simulink model "MPC_MG"  (R2020b)
settings: Solver=ode23tb  StartTime=0.0  StopTime=1  RelTol=1e-3
model workspace (MAT data in the model file):
  Ts = Simulink.Parameter
  Ts.Value = 5e-06
  Ts.DataType = 'auto'
  Ts.Dimensions = [1 1]
  secondary_on = Simulink.Parameter
  secondary_on.DataType = 'auto'
  secondary_on.Dimensions = [0 0]
values from neighbouring files (symbols this model uses):
  C_f = 50e-6    (= 5e-05)    [Four_DG_MG_PrimaryOnlyScript.m]    (also in MPC_MG_script.m; MPC_MG_script_raw_dmpc.m; MPC_MG_secondary_script.m; MPG_MG_July.m)
  f_c = 5000    [Four_DG_MG_PrimaryOnlyScript.m]    (also in MPC_MG_script.m = 40000; MPC_MG_script_raw_dmpc.m = 40000; MPC_MG_secondary_script.m = 40000; MPG_MG_July.m = 50000)
  kL = 1e-5    (= 1e-05)    [Four_DG_MG_PrimaryOnlyScript.m]    (also in MPC_MG_script.m = 1e-08; MPC_MG_script_raw_dmpc.m = 1e-08; MPC_MG_secondary_script.m = 1e-07; MPG_MG_July.m = 1e-07)
  L_f = 1.35e-3    (= 0.00135)    [Four_DG_MG_PrimaryOnlyScript.m]    (also in MPC_MG_script.m; MPC_MG_script_raw_dmpc.m; MPC_MG_secondary_script.m; MPG_MG_July.m)
  L_in1 = 0.35e-3    (= 0.00035)    [Four_DG_MG_PrimaryOnlyScript.m]    (also in MPC_MG_script.m; MPC_MG_script_raw_dmpc.m; MPC_MG_secondary_script.m; MPG_MG_July.m)
  L_in2 = 0.35e-3    (= 0.00035)    [Four_DG_MG_PrimaryOnlyScript.m]    (also in MPC_MG_script.m; MPC_MG_script_raw_dmpc.m; MPC_MG_secondary_script.m; MPG_MG_July.m)
  L_in3 = 0.35e-3    (= 0.00035)    [Four_DG_MG_PrimaryOnlyScript.m]    (also in MPC_MG_script.m; MPC_MG_script_raw_dmpc.m; MPC_MG_secondary_script.m; MPG_MG_July.m)
  L_in4 = 0.35e-3    (= 0.00035)    [Four_DG_MG_PrimaryOnlyScript.m]    (also in MPC_MG_script.m; MPC_MG_script_raw_dmpc.m; MPC_MG_secondary_script.m; MPG_MG_July.m)
  LD_ref1 = 800e-6    (= 0.0008)    [Four_DG_MG_PrimaryOnlyScript.m]    (also in MPC_MG_script.m = 0.0003; MPC_MG_script_raw_dmpc.m = 0.0003; MPC_MG_secondary_script.m = 0.0001; MPG_MG_July.m = 0.0004)
  lo_co = 0.2    [Four_DG_MG_PrimaryOnlyScript.m]    (also in MPC_MG_script.m = 0.05; MPC_MG_script_raw_dmpc.m; MPC_MG_secondary_script.m = 0.08; MPG_MG_July.m = 0.15)
  m_p1 = 9.4e-5/droopDivide    (= 9.4e-05)    [Four_DG_MG_PrimaryOnlyScript.m]    (also in MPC_MG_script.m; MPC_MG_script_raw_dmpc.m; MPC_MG_secondary_script.m; MPG_MG_July.m)
  m_p2 = 9.4e-5/droopDivide    (= 9.4e-05)    [Four_DG_MG_PrimaryOnlyScript.m]    (also in MPC_MG_script.m; MPC_MG_script_raw_dmpc.m; MPC_MG_secondary_script.m; MPG_MG_July.m)
  m_p3 = 12.5e-5/droopDivide    (= 0.000125)    [Four_DG_MG_PrimaryOnlyScript.m]    (also in MPC_MG_script.m; MPC_MG_script_raw_dmpc.m; MPC_MG_secondary_script.m; MPG_MG_July.m)
  m_p4 = 12.5e-5/droopDivide    (= 0.000125)    [Four_DG_MG_PrimaryOnlyScript.m]    (also in MPC_MG_script.m; MPC_MG_script_raw_dmpc.m; MPC_MG_secondary_script.m; MPG_MG_July.m)
  n_q1 = 1.3e-3/droopDivide2    (= 0.00013)    [Four_DG_MG_PrimaryOnlyScript.m]    (also in MPC_MG_script.m; MPC_MG_script_raw_dmpc.m; MPC_MG_secondary_script.m; MPG_MG_July.m)
  n_q2 = 1.3e-3/droopDivide2    (= 0.00013)    [Four_DG_MG_PrimaryOnlyScript.m]    (also in MPC_MG_script.m; MPC_MG_script_raw_dmpc.m; MPC_MG_secondary_script.m; MPG_MG_July.m)
  n_q3 = 1.5e-3/droopDivide2    (= 0.00015)    [Four_DG_MG_PrimaryOnlyScript.m]    (also in MPC_MG_script.m; MPC_MG_script_raw_dmpc.m; MPC_MG_secondary_script.m; MPG_MG_July.m)
  n_q4 = 1.5e-3/droopDivide2    (= 0.00015)    [Four_DG_MG_PrimaryOnlyScript.m]    (also in MPC_MG_script.m; MPC_MG_script_raw_dmpc.m; MPC_MG_secondary_script.m; MPG_MG_July.m)
  R_f = 0.1    [Four_DG_MG_PrimaryOnlyScript.m]    (also in MPC_MG_script.m; MPC_MG_script_raw_dmpc.m; MPC_MG_secondary_script.m; MPG_MG_July.m)
  R_in1 = 0.03    [Four_DG_MG_PrimaryOnlyScript.m]    (also in MPC_MG_script.m; MPC_MG_script_raw_dmpc.m; MPC_MG_secondary_script.m; MPG_MG_July.m)
  R_in2 = 0.03    [Four_DG_MG_PrimaryOnlyScript.m]    (also in MPC_MG_script.m; MPC_MG_script_raw_dmpc.m; MPC_MG_secondary_script.m; MPG_MG_July.m)
  R_in3 = 0.03    [Four_DG_MG_PrimaryOnlyScript.m]    (also in MPC_MG_script.m; MPC_MG_script_raw_dmpc.m; MPC_MG_secondary_script.m; MPG_MG_July.m)
  R_in4 = 0.03    [Four_DG_MG_PrimaryOnlyScript.m]    (also in MPC_MG_script.m; MPC_MG_script_raw_dmpc.m; MPC_MG_secondary_script.m; MPG_MG_July.m)
  Ts = 10e-6    (= 1e-05)    [Four_DG_MG_PrimaryOnlyScript.m]    (also in MPC_MG_script.m; MPC_MG_script_raw_dmpc.m; MPC_MG_secondary_script.m; MPG_MG_July.m)
  V_nom = 220*sqrt(2)    [Four_DG_MG_PrimaryOnlyScript.m]    (also in MPC_MG_script.m; MPC_MG_script_raw_dmpc.m; MPC_MG_secondary_script.m; MPG_MG_July.m)
  Vdc = 600    [Four_DG_MG_PrimaryOnlyScript.m]    (also in MPC_MG_script.m; MPC_MG_script_raw_dmpc.m; MPC_MG_secondary_script.m; MPG_MG_July.m)
  w_c_high = 2*pi*50    (= 314.159265359)    [Four_DG_MG_PrimaryOnlyScript.m]    (also in MPC_MG_script.m; MPC_MG_script_raw_dmpc.m; MPC_MG_secondary_script.m; MPG_MG_July.m)
  w_nom = 2*pi*50    (= 314.159265359)    [Four_DG_MG_PrimaryOnlyScript.m]    (also in MPC_MG_script.m; MPC_MG_script_raw_dmpc.m; MPC_MG_secondary_script.m; MPG_MG_July.m)
undefined symbols (not defined in the file or in its folder): i
libraries: powerlib x53, powerlib_meascontrol x19, eeGeneralControl x10, dspswit3 x5
(part 1 of 3)
settings Model: SimulationMode=accelerator  Creator=Linh  LastModifiedBy=Linh
settings DataIOCC: ReturnWorkspaceOutputs=off

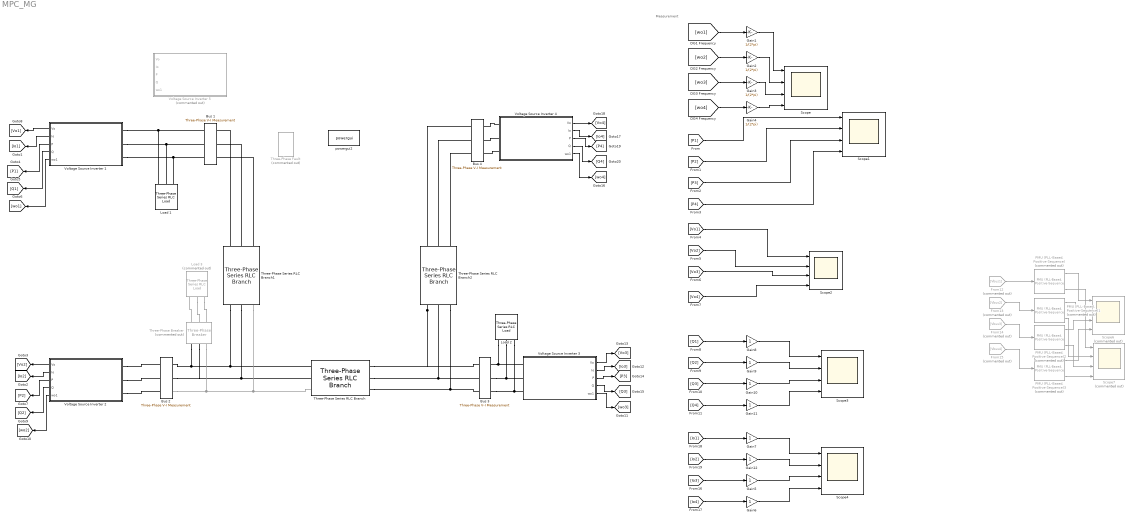
== system MPC_MG ==
  note: Measurement
  Bus 1 : powerlib/Measurements/Three-Phase V-I Measurement  VoltageMeasurement=phase-to-ground  SetLabelV=on  LabelV=Vbus1  Vpu=on  VpuLL=off  CurrentMeasurement=yes  SetLabelI=on  LabelI=Ibus1  Ipu=off  Pbase=100e6  Vbase=380  OutputType=Complex  PhasorSimulation=off  PSBequivalent=0
  Bus 2 : powerlib/Measurements/Three-Phase V-I Measurement  VoltageMeasurement=phase-to-ground  SetLabelV=on  LabelV=Vbus2  Vpu=on  VpuLL=off  CurrentMeasurement=yes  SetLabelI=on  LabelI=Ibus2  Ipu=off  Pbase=100e6  Vbase=380  OutputType=Complex  PhasorSimulation=off  PSBequivalent=0
  Bus 3 : powerlib/Measurements/Three-Phase V-I Measurement  VoltageMeasurement=phase-to-ground  SetLabelV=on  LabelV=Vbus3  Vpu=on  VpuLL=off  CurrentMeasurement=yes  SetLabelI=on  LabelI=Ibus3  Ipu=off  Pbase=100e6  Vbase=380  OutputType=Complex  PhasorSimulation=off  PSBequivalent=0
  Bus 4 : powerlib/Measurements/Three-Phase V-I Measurement  VoltageMeasurement=phase-to-phase  SetLabelV=on  LabelV=Vbus4  Vpu=off  VpuLL=on  CurrentMeasurement=no  SetLabelI=off  LabelI=Ibus4  Ipu=off  Pbase=100e6  Vbase=380  OutputType=Complex  PhasorSimulation=off  PSBequivalent=0
  From12 : From  Commented=on  GotoTag=Vbus1  TagVisibility=global
  From13 : From  Commented=on  GotoTag=Vbus2  TagVisibility=global
  From14 : From  Commented=on  GotoTag=Vbus3  TagVisibility=global
  From15 : From  Commented=on  GotoTag=Vbus4  TagVisibility=global
  Gain{1..4} (4 alike) : Gain  Gain=1/(2*pi)
  Gain{5..12} (8 alike) : Gain
  Load 1 : powerlib/Elements/Three-Phase Series RLC Load  LConnTagsString=A|B|C  Configuration=Y (grounded)  NominalVoltage=220*sqrt(3)  Vabc=[1e3 1e3 1e3]  Vabcp=[1e3 1e3 1e3]  NominalFrequency=50  UnbalancedPower=off  ActivePower=12000*3  InductivePower=12000*3  CapacitivePower=0  Pabc=[10e3 9e3 11e3]  QLabc=[100 90 110]  QCabc=[100 90 110]  Pabcp=[10e3 9e3 11e3]  QLabcp=[100 90 110]  QCabcp=[100 90 110]  Measurements=Branch voltages and currents  LoadType=constant Z
  Load 2 : powerlib/Elements/Three-Phase Series RLC Load  LConnTagsString=A|B|C  Configuration=Y (grounded)  NominalVoltage=220*sqrt(3)  Vabc=[1e3 1e3 1e3]  Vabcp=[1e3 1e3 1e3]  NominalFrequency=50  UnbalancedPower=off  ActivePower=15300*3  InductivePower=7600*3  CapacitivePower=0  Pabc=[10e3 9e3 11e3]  QLabc=[100 90 110]  QCabc=[100 90 110]  Pabcp=[10e3 9e3 11e3]  QLabcp=[100 90 110]  QCabcp=[100 90 110]  Measurements=Branch voltages and currents  LoadType=constant Z
  Load 3 : powerlib/Elements/Three-Phase Series RLC Load  Commented=on  LConnTagsString=A|B|C  Configuration=Y (grounded)  NominalVoltage=220*sqrt(3)  Vabc=[1e3 1e3 1e3]  Vabcp=[1e3 1e3 1e3]  NominalFrequency=50  UnbalancedPower=off  ActivePower=20000*3  InductivePower=12000*3  CapacitivePower=0  Pabc=[10e3 9e3 11e3]  QLabc=[100 90 110]  QCabc=[100 90 110]  Pabcp=[10e3 9e3 11e3]  QLabcp=[100 90 110]  QCabcp=[100 90 110]  Measurements=Branch voltages and currents  LoadType=constant Z
  PMU (PLL-Based, Positive-Sequence){,1..3} (4 alike) : powerlib_meascontrol/Measurements/PMU (PLL-Based, Positive-Sequence)  Commented=on  nominalFrequency=50  samplingRate=64  reportingFactor=5
      settings: SourceProductBaseCode=PS
  Scope{,1..4} (5 alike) : Scope  NumInputPorts=4
  Scope6 : Scope  Commented=on  NumInputPorts=4
  Scope7 : Scope  Commented=on  NumInputPorts=4
  Three-Phase Series RLC Branch : powerlib/Elements/Three-Phase Series RLC Branch  LConnTagsString=A|B|C  RConnTagsString=A|B|C  BranchType=RL  Resistance=0.35  Inductance=1847e-6  Capacitance=1e-6  Measurements=Branch voltages and currents
  Three-Phase Series RLC Branch1 : powerlib/Elements/Three-Phase Series RLC Branch  LConnTagsString=A|B|C  RConnTagsString=A|B|C  BranchType=RL  Resistance=0.23  Inductance=318e-6  Capacitance=1e-6  Measurements=Branch voltages and currents
  Three-Phase Series RLC Branch2 : powerlib/Elements/Three-Phase Series RLC Branch  LConnTagsString=A|B|C  RConnTagsString=A|B|C  BranchType=RL  Resistance=0.23  Inductance=318e-6  Capacitance=1e-6  Measurements=Branch voltages and currents
  Three-Phase Breaker : powerlib/Elements/Three-Phase Breaker  Commented=on  InitialState=open  SwitchA=on  SwitchB=on  SwitchC=on  SwitchTimes="[0.5  2]"  External=off  BreakerResistance=0.01  SnubberResistance=1e6  SnubberCapacitance=inf  Measurements=None
  Three-Phase Fault : powerlib/Elements/Three-Phase Fault  Commented=on  InitialStates=0  FaultA=on  FaultB=on  FaultC=off  GroundFault=off  SwitchTimes="[0.2  0.24]"  External=off  SwitchStatus=NaN  FaultResistance=0.001  GroundResistance=0.01  SnubberResistance=1e6  SnubberCapacitance=inf  Measurements=None
  Voltage Source Inverter 1 : Subsystem  mask{w_nom=w_nom, V_nom=V_nom, modT=1/f_c, m_p=m_p1, n_q=n_q1, LD_ref=LD_ref1, k_LD=kL, w_c_high=[1 w_c_high], R_f=R_f, L_f=L_f, C_f=C_f, R_in=R_in1, L_in=L_in1}
      mask prompts: w_nom "Nominal frequency (radian)"; V_nom "Nominal voltage"; modT "Sampling Time"; m_p "P-w gain"; n_q "Q-V gain"; LD_ref "Reference virtual impedance (H)"; k_LD "Virtual impedance Q gain"; w_c_high "High-pass filter denominator:"; R_f "Inductor resistance:"; L_f "Filter inductance"; C_f "Filter capacitance"; R_in "Resistance coupling"; L_in "Inductance coupling"
      mask TypeOptions w_nom: w_nom/Value
      mask TypeOptions V_nom: V_nom/Value
      mask TypeOptions modT:
      | Model Predictive Control
      | /Ts
      mask TypeOptions m_p: Droop for secondary control2/Gain5/Gain
      mask TypeOptions n_q: Droop for secondary control2/Gain4/Gain
      mask TypeOptions LD_ref: LD_ref/Value
      mask TypeOptions k_LD: k_LD/Gain
      mask TypeOptions w_c_high: High-Pass Filter/Denominator
      mask TypeOptions R_f:
      | Three-Phase
      | Series RLC Branch/Resistance
      mask TypeOptions L_f:
      | Three-Phase
      | Series RLC Branch/Inductance
      mask TypeOptions C_f:
      | Three-Phase
      | Series RLC Branch2/Capacitance
      mask TypeOptions R_in:
      | Three-Phase
      | Series RLC Branch1/Resistance
      mask TypeOptions L_in:
      | Three-Phase
      | Series RLC Branch1/Inductance
      mask DialogControl ParameterGroupVar Prompt: Microgrid-wide values
      mask DialogControl Container5 Prompt: Droop value
      mask DialogControl Container8 Prompt: Filter
  Voltage Source Inverter 2 : Subsystem  mask{w_nom=w_nom, V_nom=V_nom, modT=1/f_c, m_p=m_p2, n_q=n_q2, LD_ref=LD_ref1, k_LD=kL, w_c_high=[1 w_c_high], R_f=R_f, L_f=L_f, C_f=C_f, R_in=R_in2, L_in=L_in2}
      mask prompts: w_nom "Nominal frequency (radian)"; V_nom "Nominal voltage"; modT "Sampling Time"; m_p "P-w gain"; n_q "Q-V gain"; LD_ref "Reference virtual impedance (H)"; k_LD "Virtual impedance Q gain"; w_c_high "High-pass filter denominator:"; R_f "Inductor resistance:"; L_f "Filter inductance"; C_f "Filter capacitance"; R_in "Resistance coupling"; L_in "Inductance coupling"
      mask TypeOptions w_nom: w_nom/Value
      mask TypeOptions V_nom: V_nom/Value
      mask TypeOptions modT:
      | Model Predictive Control
      | /Ts
      mask TypeOptions m_p: Droop for secondary control2/Gain5/Gain
      mask TypeOptions n_q: Droop for secondary control2/Gain4/Gain
      mask TypeOptions LD_ref: LD_ref/Value
      mask TypeOptions k_LD: k_LD/Gain
      mask TypeOptions w_c_high: High-Pass Filter/Denominator
      mask TypeOptions R_f:
      | Three-Phase
      | Series RLC Branch/Resistance
      mask TypeOptions L_f:
      | Three-Phase
      | Series RLC Branch/Inductance
      mask TypeOptions C_f:
      | Three-Phase
      | Series RLC Branch2/Capacitance
      mask TypeOptions R_in:
      | Three-Phase
      | Series RLC Branch1/Resistance
      mask TypeOptions L_in:
      | Three-Phase
      | Series RLC Branch1/Inductance
      mask DialogControl ParameterGroupVar Prompt: Microgrid-wide values
      mask DialogControl Container5 Prompt: Droop value
      mask DialogControl Container8 Prompt: Filter
  Voltage Source Inverter 3 : Subsystem  mask{w_nom=w_nom, V_nom=V_nom, modT=1/f_c, m_p=m_p3, n_q=n_q3, LD_ref=LD_ref1, k_LD=kL, w_c_high=[1 w_c_high], R_f=R_f, L_f=L_f, C_f=C_f, R_in=R_in3, L_in=L_in3}
      mask prompts: w_nom "Nominal frequency (radian)"; V_nom "Nominal voltage"; modT "Sampling Time"; m_p "P-w gain"; n_q "Q-V gain"; LD_ref "Reference virtual impedance (H)"; k_LD "Virtual impedance Q gain"; w_c_high "High-pass filter denominator:"; R_f "Inductor resistance:"; L_f "Filter inductance"; C_f "Filter capacitance"; R_in "Resistance coupling"; L_in "Inductance coupling"
      mask TypeOptions w_nom: w_nom/Value
      mask TypeOptions V_nom: V_nom/Value
      mask TypeOptions modT:
      | Model Predictive Control
      | /Ts
      mask TypeOptions m_p: Droop for secondary control2/Gain5/Gain
      mask TypeOptions n_q: Droop for secondary control2/Gain4/Gain
      mask TypeOptions LD_ref: LD_ref/Value
      mask TypeOptions k_LD: k_LD/Gain
      mask TypeOptions w_c_high: High-Pass Filter/Denominator
      mask TypeOptions R_f:
      | Three-Phase
      | Series RLC Branch/Resistance
      mask TypeOptions L_f:
      | Three-Phase
      | Series RLC Branch/Inductance
      mask TypeOptions C_f:
      | Three-Phase
      | Series RLC Branch2/Capacitance
      mask TypeOptions R_in:
      | Three-Phase
      | Series RLC Branch1/Resistance
      mask TypeOptions L_in:
      | Three-Phase
      | Series RLC Branch1/Inductance
      mask DialogControl ParameterGroupVar Prompt: Microgrid-wide values
      mask DialogControl Container5 Prompt: Droop value
      mask DialogControl Container8 Prompt: Filter
  Voltage Source Inverter 4 : Subsystem  mask{w_nom=w_nom, V_nom=V_nom, modT=1/f_c, m_p=m_p4, n_q=n_q4, LD_ref=LD_ref1, k_LD=kL, w_c_high=[1 w_c_high], R_f=R_f, L_f=L_f, C_f=C_f, R_in=R_in4, L_in=L_in4}
      mask prompts: w_nom "Nominal frequency (radian)"; V_nom "Nominal voltage"; modT "Sampling Time"; m_p "P-w gain"; n_q "Q-V gain"; LD_ref "Reference virtual impedance (H)"; k_LD "Virtual impedance Q gain"; w_c_high "High-pass filter denominator:"; R_f "Inductor resistance:"; L_f "Filter inductance"; C_f "Filter capacitance"; R_in "Resistance coupling"; L_in "Inductance coupling"
      mask TypeOptions w_nom: w_nom/Value
      mask TypeOptions V_nom: V_nom/Value
      mask TypeOptions modT:
      | Model Predictive Control
      | /Ts
      mask TypeOptions m_p: Droop for secondary control2/Gain5/Gain
      mask TypeOptions n_q: Droop for secondary control2/Gain4/Gain
      mask TypeOptions LD_ref: LD_ref/Value
      mask TypeOptions k_LD: k_LD/Gain
      mask TypeOptions w_c_high: High-Pass Filter/Denominator
      mask TypeOptions R_f:
      | Three-Phase
      | Series RLC Branch/Resistance
      mask TypeOptions L_f:
      | Three-Phase
      | Series RLC Branch/Inductance
      mask TypeOptions C_f:
      | Three-Phase
      | Series RLC Branch2/Capacitance
      mask TypeOptions R_in:
      | Three-Phase
      | Series RLC Branch1/Resistance
      mask TypeOptions L_in:
      | Three-Phase
      | Series RLC Branch1/Inductance
      mask DialogControl ParameterGroupVar Prompt: Microgrid-wide values
      mask DialogControl Container5 Prompt: Droop value
      mask DialogControl Container8 Prompt: Filter
  Voltage Source Inverter 5 : Subsystem  Commented=on  mask{w_nom=w_nom, V_nom=V_nom, modT=1/f_c, m_p=m_p1, n_q=n_q1, LD_ref=LD_ref1, k_LD=kL, w_c_high=[1 w_c_high], R_f=R_f, L_f=L_f, C_f=C_f, R_in=R_in1, L_in=L_in1}
      mask prompts: w_nom "Nominal frequency (radian)"; V_nom "Nominal voltage"; modT "Sampling Time"; m_p "P-w gain"; n_q "Q-V gain"; LD_ref "Reference virtual impedance (H)"; k_LD "Virtual impedance Q gain"; w_c_high "High-pass filter denominator:"; R_f "Inductor resistance:"; L_f "Filter inductance"; C_f "Filter capacitance"; R_in "Resistance coupling"; L_in "Inductance coupling"
      mask TypeOptions w_nom: w_nom/Value
      mask TypeOptions V_nom: V_nom/Value
      mask TypeOptions modT:
      | Model Predictive Control
      | /Ts
      mask TypeOptions m_p: Droop for secondary control2/Gain5/Gain
      mask TypeOptions n_q: Droop for secondary control2/Gain4/Gain
      mask TypeOptions LD_ref: LD_ref/Value
      mask TypeOptions k_LD: k_LD/Gain
      mask TypeOptions w_c_high: High-Pass Filter/Denominator
      mask TypeOptions R_f:
      | Three-Phase
      | Series RLC Branch/Resistance
      mask TypeOptions L_f:
      | Three-Phase
      | Series RLC Branch/Inductance
      mask TypeOptions C_f:
      | Three-Phase
      | Series RLC Branch2/Capacitance
      mask TypeOptions R_in:
      | Three-Phase
      | Series RLC Branch1/Resistance
      mask TypeOptions L_in:
      | Three-Phase
      | Series RLC Branch1/Inductance
      mask DialogControl ParameterGroupVar Prompt: Microgrid-wide values
      mask DialogControl Container5 Prompt: Droop value
      mask DialogControl Container8 Prompt: Filter
  powergui2 : powerlib/powergui  Priority=1  SimulationMode=Discrete  SampleTime=Ts  frequency=60  Iterations=50  frequencyindice=0  Pbase=100e6  ErrMax=1e-4  UnitsV=kV  UnitsW=MW  buscounter=0  FunctionMessages=off  echomessages=off  EnableUseOfTLC=off  CurrentSourceSwitches=off  DisableSnubberDevices=off  DisableRonSwitches=off  DisableVfSwitches=off  DisplayEquations=off  AutomaticDiscreteSolvers=off  SolverType=Tustin/Backward Euler (TBE)  Interpol=off  ExternalGateDelay=off  methode=off  Ts=100  x0status=blocks  SPID=on  SwTol=0  HookPort=off  NonlinearTolerance=1e-4  nMaxIteration=100  ContinueOnMaxIteration=off  RestoreLinks=warning  ResistiveCurrentMeasurement=off  Frange=[0:2:500]  Ylog=off  Xlog=on  ShowGrid=off  save=off  variable=ZData  structure=ScopeData3  ZoomFFT=off  StartTime=0.5  cycles=1  DisplayStyle=1  fundamental=50  FreqAxis=off  MaxFrequency=1000  frequencyindicesteady=1  RmsSteady=1  display=off
  wires:
  Voltage Source Inverter 1/1(Vo) -> [Vo1]
  Voltage Source Inverter 1/2(Io) -> [Io1]
  Voltage Source Inverter 2/1(Vo) -> [Vo2]
  Voltage Source Inverter 2/2(Io) -> [Io2]
  Voltage Source Inverter 1/3(P) -> [P1]
  Voltage Source Inverter 1/4(Q) -> [Q1]
  Voltage Source Inverter 1/5(wo1) -> [wo1]
  Voltage Source Inverter 2/3(P) -> [P2]
  Voltage Source Inverter 2/4(Q) -> [Q2]
  Voltage Source Inverter 2/5(wo1) -> [wo2]
  Voltage Source Inverter 3/5(wo1) -> [wo3]
  Voltage Source Inverter 3/3(P) -> [P3]
  Voltage Source Inverter 3/1(Vo) -> [Vo3]
  Voltage Source Inverter 3/4(Q) -> [Q3]
  Voltage Source Inverter 3/2(Io) -> [Io3]
  Voltage Source Inverter 4/2(Io) -> [Io4]
  Voltage Source Inverter 4/5(wo1) -> [wo4]
  Voltage Source Inverter 4/1(Vo) -> [Vo4]
  Voltage Source Inverter 4/4(Q) -> [Q4]
  Voltage Source Inverter 4/3(P) -> [P4]
  "PMU (PLL-Based, Positive-Sequence)1"/3 -> Scope7/2
  From12/1 -> "PMU (PLL-Based, Positive-Sequence)"/1
  Gain8/1 -> Scope3/1
  Gain11/1 -> Scope3/4
  [Q4] -> Gain11/1
  [Q1] -> Gain8/1
  [wo3] -> Gain3/1
  "PMU (PLL-Based, Positive-Sequence)3"/1 -> Scope6/4
  Gain2/1 -> Scope/2
  Gain4/1 -> Scope/4
  "PMU (PLL-Based, Positive-Sequence)2"/3 -> Scope7/3
  [wo1] -> Gain1/1
  "PMU (PLL-Based, Positive-Sequence)2"/1 -> Scope6/3
  From14/1 -> "PMU (PLL-Based, Positive-Sequence)2"/1
  [P1] -> Scope1/1
  "PMU (PLL-Based, Positive-Sequence)3"/3 -> Scope7/4
  "PMU (PLL-Based, Positive-Sequence)"/1 -> Scope6/1
  "PMU (PLL-Based, Positive-Sequence)"/3 -> Scope7/1
  "PMU (PLL-Based, Positive-Sequence)1"/1 -> Scope6/2
  From13/1 -> "PMU (PLL-Based, Positive-Sequence)1"/1
  [Vo4] -> Scope2/4
  [P3] -> Scope1/3
  [Q2] -> Gain9/1
  Gain9/1 -> Scope3/2
  [P2] -> Scope1/2
  Gain3/1 -> Scope/3
  [Vo2] -> Scope2/2
  [Vo3] -> Scope2/3
  [Vo1] -> Scope2/1
  [wo2] -> Gain2/1
  [Q3] -> Gain10/1
  Gain1/1 -> Scope/1
  [P4] -> Scope1/4
  Gain10/1 -> Scope3/3
  From15/1 -> "PMU (PLL-Based, Positive-Sequence)3"/1
  [wo4] -> Gain4/1
  [Io3] -> Gain5/1
  [Io1] -> Gain7/1
  [Io2] -> Gain12/1
  Gain6/1 -> Scope4/4
  [Io4] -> Gain6/1
  Gain5/1 -> Scope4/3
  Gain7/1 -> Scope4/1
  Gain12/1 -> Scope4/2
  connections:
  Voltage Source Inverter 2/LConn1 -- Bus 2/LConn1
  Voltage Source Inverter 2/LConn2 -- Bus 2/LConn2
  Voltage Source Inverter 2/LConn3 -- Bus 2/LConn3
  Three-Phase Series RLC Branch1/RConn2 -- Three-Phase Series RLC Branch/LConn2 -- Three-Phase Breaker/LConn2 -- Bus 2/RConn2
  Bus 3/LConn2 -- Three-Phase Series RLC Branch/RConn2 -- Three-Phase Series RLC Branch2/RConn2
  Load 1/LConn3 -- Voltage Source Inverter 1/LConn3 -- Bus 1/LConn3
  Bus 2/RConn1 -- Three-Phase Series RLC Branch/LConn1 -- Three-Phase Series RLC Branch1/RConn1 -- Three-Phase Breaker/LConn1
  Three-Phase Breaker/LConn3 -- Three-Phase Series RLC Branch/LConn3 -- Three-Phase Series RLC Branch1/RConn3 -- Bus 2/RConn3
  Load 2/LConn2 -- Voltage Source Inverter 3/LConn2 -- Bus 3/RConn2
  Bus 3/LConn3 -- Three-Phase Series RLC Branch/RConn3 -- Three-Phase Series RLC Branch2/RConn3
  Load 2/LConn1 -- Voltage Source Inverter 3/LConn1 -- Bus 3/RConn1
  Load 1/LConn2 -- Voltage Source Inverter 1/LConn2 -- Bus 1/LConn2
  Three-Phase Series RLC Branch2/RConn1 -- Three-Phase Series RLC Branch/RConn1 -- Bus 3/LConn1
  Load 2/LConn3 -- Voltage Source Inverter 3/LConn3 -- Bus 3/RConn3
  Load 1/LConn1 -- Voltage Source Inverter 1/LConn1 -- Bus 1/LConn1
  Three-Phase Series RLC Branch1/LConn2 -- Bus 1/RConn2
  Load 3/LConn3 -- Three-Phase Breaker/RConn3
  Three-Phase Series RLC Branch2/LConn1 -- Bus 4/LConn1
  Three-Phase Breaker/RConn1 -- Load 3/LConn1
  Three-Phase Series RLC Branch1/LConn1 -- Bus 1/RConn1
  Three-Phase Series RLC Branch2/LConn3 -- Bus 4/LConn3
  Three-Phase Series RLC Branch2/LConn2 -- Bus 4/LConn2
  Three-Phase Series RLC Branch1/LConn3 -- Bus 1/RConn3
  Load 3/LConn2 -- Three-Phase Breaker/RConn2
  Voltage Source Inverter 4/LConn1 -- Bus 4/RConn1
  Voltage Source Inverter 4/LConn2 -- Bus 4/RConn2
  Voltage Source Inverter 4/LConn3 -- Bus 4/RConn3

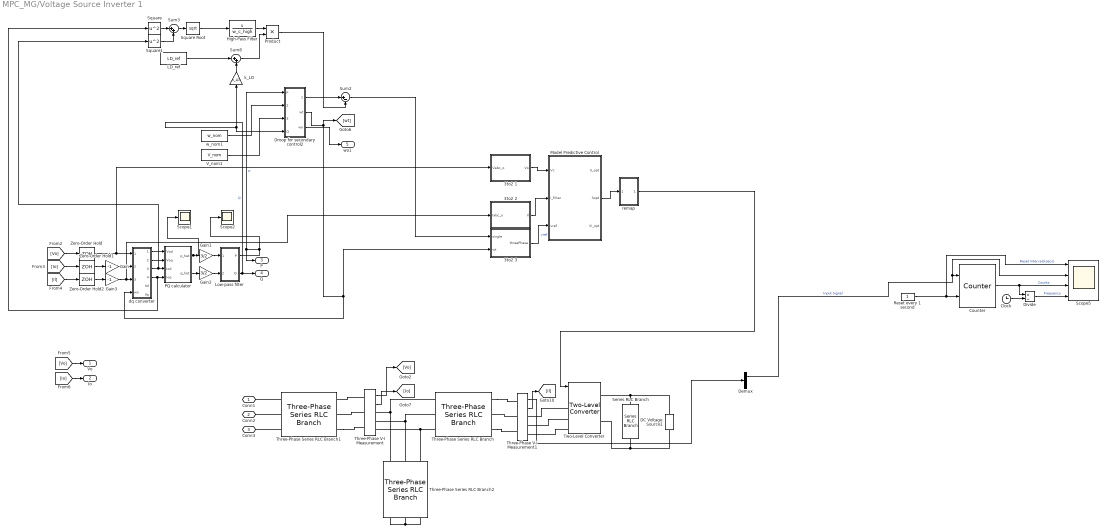
== system MPC_MG/Voltage Source Inverter 1 ==
  3to2 1 : Subsystem
  3to2 2 : Subsystem
  3to2 3 : Subsystem
  Clock : Clock
  Counter : dspswit3/Counter  Direction=Up  CountEvent=Rising edge  CounterSize=User defined  MaxCount=5e5  InitialCount=0  Output=Count  HitValue=1  ResetInput=on  SamplesPerFrame=1  Ts=1  CntDtype=double  HitDtype=Logical
  DC Voltage Source1 : powerlib/Electrical Sources/DC Voltage Source  Amplitude=Vdc  Measurements=None
  Demux : Demux  Outputs=3
  Divide : Product  Inputs=*/
  Droop for secondary control2 : Subsystem
  Gain : Gain  Gain=-1
  Gain1 : Gain  Gain=3/2
  Gain2 : Gain  Gain=3/2
  Gain3 : Gain  Gain=-1
  High-Pass Filter : TransferFcn  Numerator=[1 0]  Denominator=w_c_high
  LD_ref : Constant  Value=LD_ref
  Low-pass filter : Subsystem
  "Model Predictive Control " : MATLAB Function  TreatAsAtomicUnit=on  mask{Ts=modT, Cfilter=C_f, Lfilter=L_f, Vdc=Vdc}
      mask prompts: Ts "Sampling Time"; Cfilter "Filter Capacitor"; Lfilter "Filter Inductance"; Vdc "Input DC Voltage"
  PQ calculator : Subsystem
  Product : Product
  Reset every 1 second : Constant
  Scope1 : Scope
  Scope2 : Scope
  Scope5 : Scope  NumInputPorts=4
  Series RLC Branch : powerlib/Elements/Series RLC Branch  LConnTagsString=__new0  RConnTagsString=__new0  BranchType=RC  Resistance=30  Inductance=1e-3  SetiL0=off  InitialCurrent=0  Capacitance=80e-6  Setx0=off  InitialVoltage=0  Measurements=None
  Square : Math  Operator=square  SaturateOnIntegerOverflow=on
  Square Root : Sqrt  SaturateOnIntegerOverflow=on
  Square1 : Math  Operator=square  SaturateOnIntegerOverflow=on
  Sum2 : Sum  Inputs=|+-
  Sum3 : Sum  Inputs=|++
  Sum8 : Sum  Inputs=|++
  Three-Phase Series RLC Branch : powerlib/Elements/Three-Phase Series RLC Branch  LConnTagsString=A|B|C  RConnTagsString=A|B|C  BranchType=RL  Resistance=R_f  Inductance=L_f  Capacitance=1e-6  Measurements=None
  Three-Phase Series RLC Branch1 : powerlib/Elements/Three-Phase Series RLC Branch  LConnTagsString=A|B|C  RConnTagsString=A|B|C  BranchType=RL  Resistance=R_in  Inductance=L_in  Capacitance=1e-6  Measurements=None
  Three-Phase Series RLC Branch2 : powerlib/Elements/Three-Phase Series RLC Branch  LConnTagsString=A|B|C  RConnTagsString=A|B|C  BranchType=C  Resistance=R_f  Inductance=1e-3  Capacitance=C_f  Measurements=None
  Three-Phase V-I Measurement : powerlib/Measurements/Three-Phase V-I Measurement  VoltageMeasurement=phase-to-ground  SetLabelV=off  LabelV=Vo1  Vpu=off  VpuLL=off  CurrentMeasurement=yes  SetLabelI=off  LabelI=Io1  Ipu=off  Pbase=100e6  Vbase=500e3  OutputType=Complex  PhasorSimulation=off  PSBequivalent=0
  Three-Phase V-I Measurement1 : powerlib/Measurements/Three-Phase V-I Measurement  VoltageMeasurement=phase-to-ground  SetLabelV=off  LabelV=Vl2  Vpu=off  VpuLL=off  CurrentMeasurement=yes  SetLabelI=off  LabelI=Il2  Ipu=off  Pbase=100e6  Vbase=500e3  OutputType=Complex  PhasorSimulation=off  PSBequivalent=0
  Two-Level Converter : powerlib/Power Electronics/Two-Level Converter  ModelType=Switching devices  Ron=1e-3  Rs=1e6  Cs=inf  Vforward=[0,0]  Ron_Diode=1e-3  Rs_Diode=1e6  Cs_Diode=inf  Vf_Diode=1e-3  Rs_CurrentSource=inf
      settings: SourceProductBaseCode=PS
  V_nom1 : Constant  Value=V_nom
  Zero-Order Hold : ZeroOrderHold  SampleTime=modT
  Zero-Order Hold1 : ZeroOrderHold  SampleTime=modT
  Zero-Order Hold2 : ZeroOrderHold  SampleTime=modT
  dq converter : Subsystem
  k_LD : Gain  Gain=k_LD
  remap : Subsystem
  w_nom1 : Constant  Value=w_nom
  Conn1 : PMIOPort  Side=Left
  Conn2 : PMIOPort  Port=2  Side=Left
  Conn3 : PMIOPort  Port=3  Side=Left
  Vo : Outport
  Io : Outport  Port=2
  P : Outport  Port=3
  Q : Outport  Port=4
  wo1 : Outport  Port=5
  wires:
  Gain/1 -> dq converter/2(Iodq)
  Droop for secondary control2/2(wt) -> [wt], dq converter/4(wo), 3to2 3/2("wt ")
  Gain2/1 -> Low-pass filter/2(q_hat)
  PQ calculator/2(q_hat) -> Gain2/1
  Gain1/1 -> Low-pass filter/1(p_hat)
  dq converter/2(Voq) -> PQ calculator/2(Voq)
  [Il] -> Zero-Order Hold2/1
  PQ calculator/1(p_hat) -> Scope1/1, Gain1/1
  [Io] -> Zero-Order Hold1/1
  dq converter/1(Vod) -> PQ calculator/1(Vod)
  [Vo] -> Vo/1
  [Io] -> Io/1
  Three-Phase V-I Measurement/1 -> [Vo]
  Three-Phase V-I Measurement/2 -> [Io]
  Three-Phase V-I Measurement1/2 -> [Il]
  3to2 1/1(Vo) -> "Model Predictive Control "/1(Vc)
  3to2 3/1(threePhase) -> "Model Predictive Control "/3(vref)  "vref"
  3to2 2/1(Il) -> "Model Predictive Control "/2(i_filter)
  [Vo] -> Zero-Order Hold/1
  "Model Predictive Control "/2(Sopt) -> remap/1(In1)
  Gain3/1 -> 3to2 2/1("Iabc_o "), dq converter/3(Ildq)
  remap/1(Out1) -> Two-Level Converter/1
  Zero-Order Hold/1 -> 3to2 1/1("Vabc_o "), dq converter/1(Vodq)
  Zero-Order Hold1/1 -> Gain/1
  Zero-Order Hold2/1 -> Gain3/1
  Sum2/1 -> 3to2 3/1("single ")
  Three-Phase V-I Measurement1/1 -> Demux/1
  Demux/1 -> Counter/1, Scope5/2  "Input Signal"
  Clock/1 -> Divide/2
  Reset every 1 second/1 -> Scope5/1, Counter/2  "Reset Intervals(secs)"
  Counter/1 -> Scope5/3, Divide/1  "Counts"
  Divide/1 -> Scope5/4  "Frequency"
  w_nom1/1 -> Droop for secondary control2/2(w_nom)
  V_nom1/1 -> Droop for secondary control2/3(V_nom)
  Square1/1 -> Sum3/2
  Sum3/1 -> Square Root/1
  Sum8/1 -> Product/2
  k_LD/1 -> Sum8/2
  Square Root/1 -> High-Pass Filter/1
  Low-pass filter/2(Q) -> Q/1, Droop for secondary control2/4(Q), k_LD/1  "Q"
  Droop for secondary control2/1(Vref) -> Sum2/1
  LD_ref/1 -> Sum8/1
  dq converter/3(Iod) -> Square1/1, PQ calculator/3(Iod)
  Droop for secondary control2/3(wo) -> wo1/1
  Product/1 -> Sum2/2
  dq converter/4(Ioq) -> Square/1, PQ calculator/4(Ioq)
  High-Pass Filter/1 -> Product/1
  Low-pass filter/1(P) -> Scope2/1, P/1, Droop for secondary control2/1(P)  "P"
  Square/1 -> Sum3/1
  connections:
  Three-Phase Series RLC Branch2/LConn1 -- Three-Phase V-I Measurement/RConn1 -- Three-Phase Series RLC Branch/LConn1
  Two-Level Converter/RConn1 -- DC Voltage Source1/RConn1 -- Series RLC Branch/LConn1
  Three-Phase Series RLC Branch2/RConn3 -- Three-Phase Series RLC Branch2/RConn1 -- Three-Phase Series RLC Branch2/RConn2
  Three-Phase Series RLC Branch2/LConn3 -- Three-Phase Series RLC Branch/LConn3 -- Three-Phase V-I Measurement/RConn3
  Two-Level Converter/RConn2 -- Series RLC Branch/RConn1 -- DC Voltage Source1/LConn1
  Three-Phase Series RLC Branch/LConn2 -- Three-Phase V-I Measurement/RConn2 -- Three-Phase Series RLC Branch2/LConn2
  Two-Level Converter/LConn1 -- Three-Phase V-I Measurement1/RConn1
  Three-Phase V-I Measurement1/LConn2 -- Three-Phase Series RLC Branch/RConn2
  Two-Level Converter/LConn2 -- Three-Phase V-I Measurement1/RConn2
  Three-Phase Series RLC Branch1/LConn2 -- Conn2/RConn1
  Two-Level Converter/LConn3 -- Three-Phase V-I Measurement1/RConn3
  Three-Phase Series RLC Branch/RConn1 -- Three-Phase V-I Measurement1/LConn1
  Three-Phase Series RLC Branch1/LConn3 -- Conn3/RConn1
  Three-Phase V-I Measurement/LConn1 -- Three-Phase Series RLC Branch1/RConn1
  Three-Phase Series RLC Branch1/LConn1 -- Conn1/RConn1
  Three-Phase V-I Measurement/LConn2 -- Three-Phase Series RLC Branch1/RConn2
  Three-Phase Series RLC Branch1/RConn3 -- Three-Phase V-I Measurement/LConn3
  Three-Phase Series RLC Branch/RConn3 -- Three-Phase V-I Measurement1/LConn3

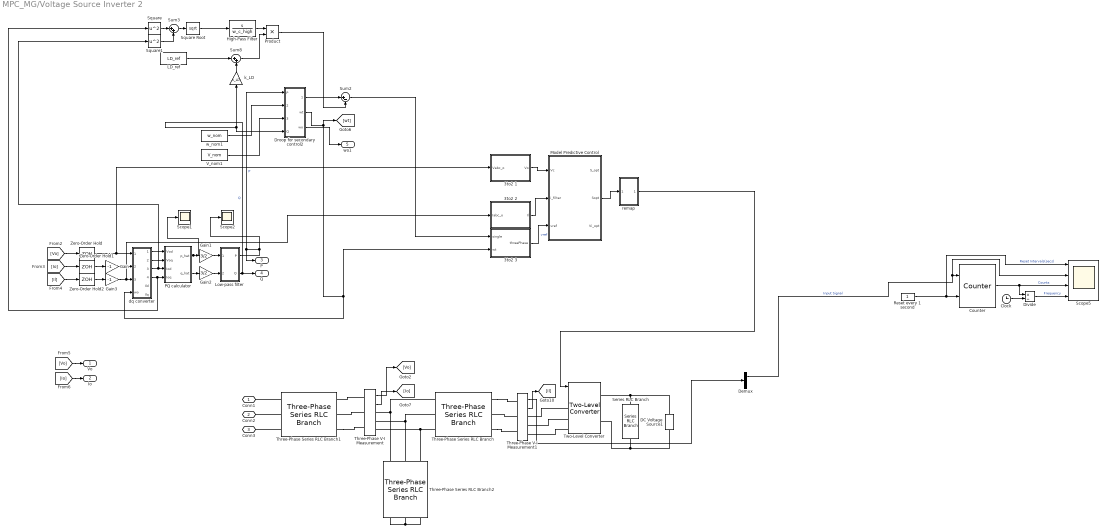
== system MPC_MG/Voltage Source Inverter 2 ==
  3to2 1 : Subsystem
  3to2 2 : Subsystem
  3to2 3 : Subsystem
  Clock : Clock
  Counter : dspswit3/Counter  Direction=Up  CountEvent=Rising edge  CounterSize=User defined  MaxCount=5e5  InitialCount=0  Output=Count  HitValue=1  ResetInput=on  SamplesPerFrame=1  Ts=1  CntDtype=double  HitDtype=Logical
  DC Voltage Source1 : powerlib/Electrical Sources/DC Voltage Source  Amplitude=Vdc  Measurements=None
  Demux : Demux  Outputs=3
  Divide : Product  Inputs=*/
  Droop for secondary control2 : Subsystem
  Gain : Gain  Gain=-1
  Gain1 : Gain  Gain=3/2
  Gain2 : Gain  Gain=3/2
  Gain3 : Gain  Gain=-1
  High-Pass Filter : TransferFcn  Numerator=[1 0]  Denominator=w_c_high
  LD_ref : Constant  Value=LD_ref
  Low-pass filter : Subsystem
  "Model Predictive Control " : MATLAB Function  TreatAsAtomicUnit=on  mask{Ts=modT, Cfilter=C_f, Lfilter=L_f, Vdc=Vdc}
      mask prompts: Ts "Sampling Time"; Cfilter "Filter Capacitor"; Lfilter "Filter Inductance"; Vdc "Input DC Voltage"
  PQ calculator : Subsystem
  Product : Product
  Reset every 1 second : Constant
  Scope1 : Scope
  Scope2 : Scope
  Scope5 : Scope  NumInputPorts=4
  Series RLC Branch : powerlib/Elements/Series RLC Branch  LConnTagsString=__new0  RConnTagsString=__new0  BranchType=RC  Resistance=30  Inductance=1e-3  SetiL0=off  InitialCurrent=0  Capacitance=80e-6  Setx0=off  InitialVoltage=0  Measurements=None
  Square : Math  Operator=square  SaturateOnIntegerOverflow=on
  Square Root : Sqrt  SaturateOnIntegerOverflow=on
  Square1 : Math  Operator=square  SaturateOnIntegerOverflow=on
  Sum2 : Sum  Inputs=|+-
  Sum3 : Sum  Inputs=|++
  Sum8 : Sum  Inputs=|++
  Three-Phase Series RLC Branch : powerlib/Elements/Three-Phase Series RLC Branch  LConnTagsString=A|B|C  RConnTagsString=A|B|C  BranchType=RL  Resistance=R_f  Inductance=L_f  Capacitance=1e-6  Measurements=None
  Three-Phase Series RLC Branch1 : powerlib/Elements/Three-Phase Series RLC Branch  LConnTagsString=A|B|C  RConnTagsString=A|B|C  BranchType=RL  Resistance=R_in  Inductance=L_in  Capacitance=1e-6  Measurements=None
  Three-Phase Series RLC Branch2 : powerlib/Elements/Three-Phase Series RLC Branch  LConnTagsString=A|B|C  RConnTagsString=A|B|C  BranchType=C  Resistance=R_f  Inductance=1e-3  Capacitance=C_f  Measurements=None
  Three-Phase V-I Measurement : powerlib/Measurements/Three-Phase V-I Measurement  VoltageMeasurement=phase-to-ground  SetLabelV=off  LabelV=Vo1  Vpu=off  VpuLL=off  CurrentMeasurement=yes  SetLabelI=off  LabelI=Io1  Ipu=off  Pbase=100e6  Vbase=500e3  OutputType=Complex  PhasorSimulation=off  PSBequivalent=0
  Three-Phase V-I Measurement1 : powerlib/Measurements/Three-Phase V-I Measurement  VoltageMeasurement=phase-to-ground  SetLabelV=off  LabelV=Vl2  Vpu=off  VpuLL=off  CurrentMeasurement=yes  SetLabelI=off  LabelI=Il2  Ipu=off  Pbase=100e6  Vbase=500e3  OutputType=Complex  PhasorSimulation=off  PSBequivalent=0
  Two-Level Converter : powerlib/Power Electronics/Two-Level Converter  ModelType=Switching devices  Ron=1e-3  Rs=1e6  Cs=inf  Vforward=[0,0]  Ron_Diode=1e-3  Rs_Diode=1e6  Cs_Diode=inf  Vf_Diode=1e-3  Rs_CurrentSource=inf
      settings: SourceProductBaseCode=PS
  V_nom1 : Constant  Value=V_nom
  Zero-Order Hold : ZeroOrderHold  SampleTime=modT
  Zero-Order Hold1 : ZeroOrderHold  SampleTime=modT
  Zero-Order Hold2 : ZeroOrderHold  SampleTime=modT
  dq converter : Subsystem
  k_LD : Gain  Gain=k_LD
  remap : Subsystem
  w_nom1 : Constant  Value=w_nom
  Conn1 : PMIOPort  Side=Left
  Conn2 : PMIOPort  Port=2  Side=Left
  Conn3 : PMIOPort  Port=3  Side=Left
  Vo : Outport
  Io : Outport  Port=2
  P : Outport  Port=3
  Q : Outport  Port=4
  wo1 : Outport  Port=5
  wires:
  Gain/1 -> dq converter/2(Iodq)
  Droop for secondary control2/2(wt) -> [wt], dq converter/4(wo), 3to2 3/2("wt ")
  Gain2/1 -> Low-pass filter/2(q_hat)
  PQ calculator/2(q_hat) -> Gain2/1
  Gain1/1 -> Low-pass filter/1(p_hat)
  dq converter/2(Voq) -> PQ calculator/2(Voq)
  [Il] -> Zero-Order Hold2/1
  PQ calculator/1(p_hat) -> Scope1/1, Gain1/1
  [Io] -> Zero-Order Hold1/1
  dq converter/1(Vod) -> PQ calculator/1(Vod)
  [Vo] -> Vo/1
  [Io] -> Io/1
  Three-Phase V-I Measurement/1 -> [Vo]
  Three-Phase V-I Measurement/2 -> [Io]
  Three-Phase V-I Measurement1/2 -> [Il]
  3to2 1/1(Vo) -> "Model Predictive Control "/1(Vc)
  3to2 3/1(threePhase) -> "Model Predictive Control "/3(vref)  "vref"
  3to2 2/1(Il) -> "Model Predictive Control "/2(i_filter)
  [Vo] -> Zero-Order Hold/1
  "Model Predictive Control "/2(Sopt) -> remap/1(In1)
  Gain3/1 -> 3to2 2/1("Iabc_o "), dq converter/3(Ildq)
  remap/1(Out1) -> Two-Level Converter/1
  Zero-Order Hold/1 -> 3to2 1/1("Vabc_o "), dq converter/1(Vodq)
  Zero-Order Hold1/1 -> Gain/1
  Zero-Order Hold2/1 -> Gain3/1
  Sum2/1 -> 3to2 3/1("single ")
  Three-Phase V-I Measurement1/1 -> Demux/1
  Demux/1 -> Counter/1, Scope5/2  "Input Signal"
  Clock/1 -> Divide/2
  Reset every 1 second/1 -> Scope5/1, Counter/2  "Reset Intervals(secs)"
  Counter/1 -> Scope5/3, Divide/1  "Counts"
  Divide/1 -> Scope5/4  "Frequency"
  w_nom1/1 -> Droop for secondary control2/2(w_nom)
  V_nom1/1 -> Droop for secondary control2/3(V_nom)
  Square1/1 -> Sum3/2
  Sum3/1 -> Square Root/1
  Sum8/1 -> Product/2
  k_LD/1 -> Sum8/2
  Square Root/1 -> High-Pass Filter/1
  Low-pass filter/2(Q) -> Q/1, Droop for secondary control2/4(Q), k_LD/1  "Q"
  Droop for secondary control2/1(Vref) -> Sum2/1
  LD_ref/1 -> Sum8/1
  dq converter/3(Iod) -> Square1/1, PQ calculator/3(Iod)
  Droop for secondary control2/3(wo) -> wo1/1
  Product/1 -> Sum2/2
  dq converter/4(Ioq) -> Square/1, PQ calculator/4(Ioq)
  High-Pass Filter/1 -> Product/1
  Low-pass filter/1(P) -> Scope2/1, P/1, Droop for secondary control2/1(P)  "P"
  Square/1 -> Sum3/1
  connections:
  Three-Phase Series RLC Branch2/LConn1 -- Three-Phase V-I Measurement/RConn1 -- Three-Phase Series RLC Branch/LConn1
  Two-Level Converter/RConn1 -- DC Voltage Source1/RConn1 -- Series RLC Branch/LConn1
  Three-Phase Series RLC Branch2/RConn3 -- Three-Phase Series RLC Branch2/RConn1 -- Three-Phase Series RLC Branch2/RConn2
  Three-Phase Series RLC Branch2/LConn3 -- Three-Phase Series RLC Branch/LConn3 -- Three-Phase V-I Measurement/RConn3
  Two-Level Converter/RConn2 -- Series RLC Branch/RConn1 -- DC Voltage Source1/LConn1
  Three-Phase Series RLC Branch/LConn2 -- Three-Phase V-I Measurement/RConn2 -- Three-Phase Series RLC Branch2/LConn2
  Two-Level Converter/LConn1 -- Three-Phase V-I Measurement1/RConn1
  Three-Phase V-I Measurement1/LConn2 -- Three-Phase Series RLC Branch/RConn2
  Two-Level Converter/LConn2 -- Three-Phase V-I Measurement1/RConn2
  Three-Phase Series RLC Branch1/LConn2 -- Conn2/RConn1
  Two-Level Converter/LConn3 -- Three-Phase V-I Measurement1/RConn3
  Three-Phase Series RLC Branch/RConn1 -- Three-Phase V-I Measurement1/LConn1
  Three-Phase Series RLC Branch1/LConn3 -- Conn3/RConn1
  Three-Phase V-I Measurement/LConn1 -- Three-Phase Series RLC Branch1/RConn1
  Three-Phase Series RLC Branch1/LConn1 -- Conn1/RConn1
  Three-Phase V-I Measurement/LConn2 -- Three-Phase Series RLC Branch1/RConn2
  Three-Phase Series RLC Branch1/RConn3 -- Three-Phase V-I Measurement/LConn3
  Three-Phase Series RLC Branch/RConn3 -- Three-Phase V-I Measurement1/LConn3

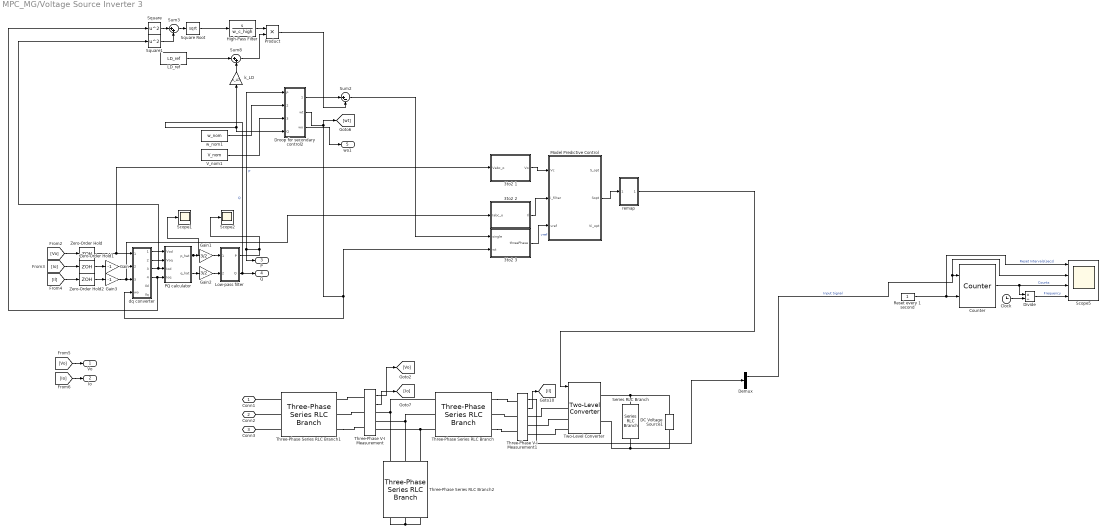
== system MPC_MG/Voltage Source Inverter 3 ==
  3to2 1 : Subsystem
  3to2 2 : Subsystem
  3to2 3 : Subsystem
  Clock : Clock
  Counter : dspswit3/Counter  Direction=Up  CountEvent=Rising edge  CounterSize=User defined  MaxCount=5e5  InitialCount=0  Output=Count  HitValue=1  ResetInput=on  SamplesPerFrame=1  Ts=1  CntDtype=double  HitDtype=Logical
  DC Voltage Source1 : powerlib/Electrical Sources/DC Voltage Source  Amplitude=Vdc  Measurements=None
  Demux : Demux  Outputs=3
  Divide : Product  Inputs=*/
  Droop for secondary control2 : Subsystem
  Gain : Gain  Gain=-1
  Gain1 : Gain  Gain=3/2
  Gain2 : Gain  Gain=3/2
  Gain3 : Gain  Gain=-1
  High-Pass Filter : TransferFcn  Numerator=[1 0]  Denominator=w_c_high
  LD_ref : Constant  Value=LD_ref
  Low-pass filter : Subsystem
  "Model Predictive Control " : MATLAB Function  TreatAsAtomicUnit=on  mask{Ts=modT, Cfilter=C_f, Lfilter=L_f, Vdc=Vdc}
      mask prompts: Ts "Sampling Time"; Cfilter "Filter Capacitor"; Lfilter "Filter Inductance"; Vdc "Input DC Voltage"
  PQ calculator : Subsystem
  Product : Product
  Reset every 1 second : Constant
  Scope1 : Scope
  Scope2 : Scope
  Scope5 : Scope  NumInputPorts=4
  Series RLC Branch : powerlib/Elements/Series RLC Branch  LConnTagsString=__new0  RConnTagsString=__new0  BranchType=RC  Resistance=30  Inductance=1e-3  SetiL0=off  InitialCurrent=0  Capacitance=80e-6  Setx0=off  InitialVoltage=0  Measurements=None
  Square : Math  Operator=square  SaturateOnIntegerOverflow=on
  Square Root : Sqrt  SaturateOnIntegerOverflow=on
  Square1 : Math  Operator=square  SaturateOnIntegerOverflow=on
  Sum2 : Sum  Inputs=|+-
  Sum3 : Sum  Inputs=|++
  Sum8 : Sum  Inputs=|++
  Three-Phase Series RLC Branch : powerlib/Elements/Three-Phase Series RLC Branch  LConnTagsString=A|B|C  RConnTagsString=A|B|C  BranchType=RL  Resistance=R_f  Inductance=L_f  Capacitance=1e-6  Measurements=None
  Three-Phase Series RLC Branch1 : powerlib/Elements/Three-Phase Series RLC Branch  LConnTagsString=A|B|C  RConnTagsString=A|B|C  BranchType=RL  Resistance=R_in  Inductance=L_in  Capacitance=1e-6  Measurements=None
  Three-Phase Series RLC Branch2 : powerlib/Elements/Three-Phase Series RLC Branch  LConnTagsString=A|B|C  RConnTagsString=A|B|C  BranchType=C  Resistance=R_f  Inductance=1e-3  Capacitance=C_f  Measurements=None
  Three-Phase V-I Measurement : powerlib/Measurements/Three-Phase V-I Measurement  VoltageMeasurement=phase-to-ground  SetLabelV=off  LabelV=Vo1  Vpu=off  VpuLL=off  CurrentMeasurement=yes  SetLabelI=off  LabelI=Io1  Ipu=off  Pbase=100e6  Vbase=500e3  OutputType=Complex  PhasorSimulation=off  PSBequivalent=0
  Three-Phase V-I Measurement1 : powerlib/Measurements/Three-Phase V-I Measurement  VoltageMeasurement=phase-to-ground  SetLabelV=off  LabelV=Vl2  Vpu=off  VpuLL=off  CurrentMeasurement=yes  SetLabelI=off  LabelI=Il2  Ipu=off  Pbase=100e6  Vbase=500e3  OutputType=Complex  PhasorSimulation=off  PSBequivalent=0
  Two-Level Converter : powerlib/Power Electronics/Two-Level Converter  ModelType=Switching devices  Ron=1e-3  Rs=1e6  Cs=inf  Vforward=[0,0]  Ron_Diode=1e-3  Rs_Diode=1e6  Cs_Diode=inf  Vf_Diode=1e-3  Rs_CurrentSource=inf
      settings: SourceProductBaseCode=PS
  V_nom1 : Constant  Value=V_nom
  Zero-Order Hold : ZeroOrderHold  SampleTime=modT
  Zero-Order Hold1 : ZeroOrderHold  SampleTime=modT
  Zero-Order Hold2 : ZeroOrderHold  SampleTime=modT
  dq converter : Subsystem
  k_LD : Gain  Gain=k_LD
  remap : Subsystem
  w_nom1 : Constant  Value=w_nom
  Conn1 : PMIOPort  Side=Left
  Conn2 : PMIOPort  Port=2  Side=Left
  Conn3 : PMIOPort  Port=3  Side=Left
  Vo : Outport
  Io : Outport  Port=2
  P : Outport  Port=3
  Q : Outport  Port=4
  wo1 : Outport  Port=5
  wires:
  Gain/1 -> dq converter/2(Iodq)
  Droop for secondary control2/2(wt) -> [wt], dq converter/4(wo), 3to2 3/2("wt ")
  Gain2/1 -> Low-pass filter/2(q_hat)
  PQ calculator/2(q_hat) -> Gain2/1
  Gain1/1 -> Low-pass filter/1(p_hat)
  dq converter/2(Voq) -> PQ calculator/2(Voq)
  [Il] -> Zero-Order Hold2/1
  PQ calculator/1(p_hat) -> Scope1/1, Gain1/1
  [Io] -> Zero-Order Hold1/1
  dq converter/1(Vod) -> PQ calculator/1(Vod)
  [Vo] -> Vo/1
  [Io] -> Io/1
  Three-Phase V-I Measurement/1 -> [Vo]
  Three-Phase V-I Measurement/2 -> [Io]
  Three-Phase V-I Measurement1/2 -> [Il]
  3to2 1/1(Vo) -> "Model Predictive Control "/1(Vc)
  3to2 3/1(threePhase) -> "Model Predictive Control "/3(vref)  "vref"
  3to2 2/1(Il) -> "Model Predictive Control "/2(i_filter)
  [Vo] -> Zero-Order Hold/1
  "Model Predictive Control "/2(Sopt) -> remap/1(In1)
  Gain3/1 -> 3to2 2/1("Iabc_o "), dq converter/3(Ildq)
  remap/1(Out1) -> Two-Level Converter/1
  Zero-Order Hold/1 -> 3to2 1/1("Vabc_o "), dq converter/1(Vodq)
  Zero-Order Hold1/1 -> Gain/1
  Zero-Order Hold2/1 -> Gain3/1
  Sum2/1 -> 3to2 3/1("single ")
  Three-Phase V-I Measurement1/1 -> Demux/1
  Demux/1 -> Counter/1, Scope5/2  "Input Signal"
  Clock/1 -> Divide/2
  Reset every 1 second/1 -> Scope5/1, Counter/2  "Reset Intervals(secs)"
  Counter/1 -> Scope5/3, Divide/1  "Counts"
  Divide/1 -> Scope5/4  "Frequency"
  w_nom1/1 -> Droop for secondary control2/2(w_nom)
  V_nom1/1 -> Droop for secondary control2/3(V_nom)
  Square1/1 -> Sum3/2
  Sum3/1 -> Square Root/1
  Sum8/1 -> Product/2
  k_LD/1 -> Sum8/2
  Square Root/1 -> High-Pass Filter/1
  Low-pass filter/2(Q) -> Q/1, Droop for secondary control2/4(Q), k_LD/1  "Q"
  Droop for secondary control2/1(Vref) -> Sum2/1
  LD_ref/1 -> Sum8/1
  dq converter/3(Iod) -> Square1/1, PQ calculator/3(Iod)
  Droop for secondary control2/3(wo) -> wo1/1
  Product/1 -> Sum2/2
  dq converter/4(Ioq) -> Square/1, PQ calculator/4(Ioq)
  High-Pass Filter/1 -> Product/1
  Low-pass filter/1(P) -> Scope2/1, P/1, Droop for secondary control2/1(P)  "P"
  Square/1 -> Sum3/1
  connections:
  Three-Phase Series RLC Branch2/LConn1 -- Three-Phase V-I Measurement/RConn1 -- Three-Phase Series RLC Branch/LConn1
  Two-Level Converter/RConn1 -- DC Voltage Source1/RConn1 -- Series RLC Branch/LConn1
  Three-Phase Series RLC Branch2/RConn3 -- Three-Phase Series RLC Branch2/RConn1 -- Three-Phase Series RLC Branch2/RConn2
  Three-Phase Series RLC Branch2/LConn3 -- Three-Phase Series RLC Branch/LConn3 -- Three-Phase V-I Measurement/RConn3
  Two-Level Converter/RConn2 -- Series RLC Branch/RConn1 -- DC Voltage Source1/LConn1
  Three-Phase Series RLC Branch/LConn2 -- Three-Phase V-I Measurement/RConn2 -- Three-Phase Series RLC Branch2/LConn2
  Two-Level Converter/LConn1 -- Three-Phase V-I Measurement1/RConn1
  Three-Phase V-I Measurement1/LConn2 -- Three-Phase Series RLC Branch/RConn2
  Two-Level Converter/LConn2 -- Three-Phase V-I Measurement1/RConn2
  Three-Phase Series RLC Branch1/LConn2 -- Conn2/RConn1
  Two-Level Converter/LConn3 -- Three-Phase V-I Measurement1/RConn3
  Three-Phase Series RLC Branch/RConn1 -- Three-Phase V-I Measurement1/LConn1
  Three-Phase Series RLC Branch1/LConn3 -- Conn3/RConn1
  Three-Phase V-I Measurement/LConn1 -- Three-Phase Series RLC Branch1/RConn1
  Three-Phase Series RLC Branch1/LConn1 -- Conn1/RConn1
  Three-Phase V-I Measurement/LConn2 -- Three-Phase Series RLC Branch1/RConn2
  Three-Phase Series RLC Branch1/RConn3 -- Three-Phase V-I Measurement/LConn3
  Three-Phase Series RLC Branch/RConn3 -- Three-Phase V-I Measurement1/LConn3
